simulink model "velocity_pi_pid_control"  (R2025a)
settings: Solver=ode3  StartTime=0.0  StopTime=10  FixedStep=ts  RelTol=1e-3  EnableMultiTasking=on
undefined symbols (not defined in the file): DiscIntNeverNeededParam, ts
libraries: arduinolib x3, simulink x2, arduinosensorlib x1, dspstat3 x1, dspsrcs4 x1
settings Model: SILPILModeSetting=veronly  ExtModeTrigDuration=2  Creator=tsuga  LastModifiedBy=ANUSHKA
settings SolverCC: AutoInsertRateTranBlk=on
settings DataIOCC: SaveOutput=off  SignalLogging=off  DSMLogging=off  SaveTime=off  ReturnWorkspaceOutputs=off
settings OptimizationCC: StrengthReduction=on  PassReuseOutputArgsAs=Individual arguments  ZeroExternalMemoryAtStartup=off  ZeroInternalMemoryAtStartup=off  MaxStackSize=64  OptimizeBlockOrder=speed  OptimizationPriority=Speed  OptimizationCustomize=off  MultiThreadedLoops=on  AutoScheduleForLoops=on  EfficientTunableParamExpr=on
settings DebuggingCC: ParameterTunabilityLossMsg=error  UnconnectedInputMsg=warning  UnconnectedOutputMsg=warning  UnconnectedLineMsg=warning
settings HardwareCC: ProdBitPerInt=16.0  ProdBitPerPointer=16.0  ProdBitPerSizeT=16.0  ProdBitPerPtrDiffT=16.0  ProdLargestAtomicFloat=None  ProdWordSize=8.0  ProdHWDeviceType=Atmel->AVR
settings ModelReferenceCC: EnableRefExpFcnMdlSchedulingChecks=on
settings SFSimCC: MATLABDynamicMemAlloc=off
settings RTWCC: SystemTargetFile=ert.tlc  HardwareBoard=Arduino Uno  TemplateMakefile=ert_default_tmf  Toolchain=Arduino AVR  BuildConfiguration=Faster Runs  GPUComputeCapability=3.5  DLArmComputeVersion=19.05  Description=Embedded Coder
settings CodeAppCC: ForceParamTrailComments=on  IgnoreCustomStorageClasses=off  OperatorAnnotations=on  SimulinkDataObjDesc=on  SFDataObjDesc=on  InsertBlockDesc=on
settings ERTTargetCC: ExtModeTransport=3.0  ExtModeAutomaticAllocSize=off  ExtModeStaticAllocSize=250.0  InlinedParameterPlacement=Hierarchical  DynamicArrayContainerType=coder::array  SupportContinuousTime=on  SupportVariableSizeSignals=on

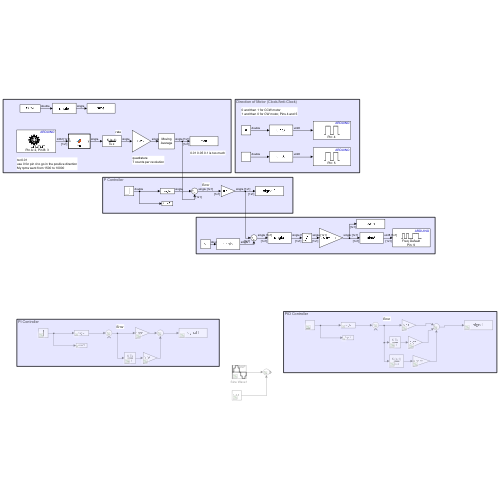
[thumbnail: Simulink's stored preview of the top-level diagram]
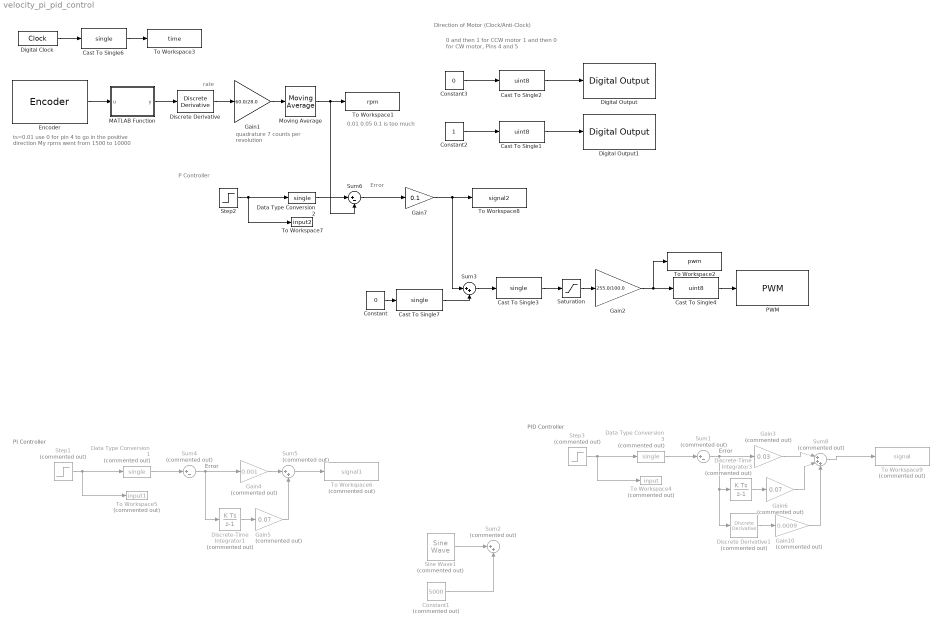
== system velocity_pi_pid_control ==
  note: Direction of Motor (Clock/Anti-Clock)
  note: 0.01 0.05 0.1 is too much
  note: rate
  note: quadrature
      | 7 counts per revolution
  note: ts=0.01
      | use 0 for pin 4 to go in the positive direction
      | My rpms went from 1500 to 10000
  note: 0 and then 1 for CCW motor
      | 1 and then 0 for CW motor, Pins 4 and 5
  note: PI Controller
  note: Error
  note: P Controller
  note: Error
  note: PID Controller
  note: Error
  Cast To Single1 : DataTypeConversion  OutDataTypeStr=uint8  SaturateOnIntegerOverflow=off  RndMeth=Floor
  Cast To Single2 : DataTypeConversion  OutDataTypeStr=uint8  SaturateOnIntegerOverflow=off  RndMeth=Floor
  Cast To Single3 : DataTypeConversion  OutDataTypeStr=single  SaturateOnIntegerOverflow=off  RndMeth=Floor
  Cast To Single4 : DataTypeConversion  OutDataTypeStr=uint8  SaturateOnIntegerOverflow=off  RndMeth=Floor
  Cast To Single6 : DataTypeConversion  OutDataTypeStr=single  SaturateOnIntegerOverflow=off  RndMeth=Floor
  Cast To Single7 : DataTypeConversion  OutDataTypeStr=single  SaturateOnIntegerOverflow=off  RndMeth=Floor
  Constant : Constant  Value=0  SampleTime=ts
  Constant1 : Constant  Commented=on  Value=5000  OutDataTypeStr=double
  Constant2 : Constant  SampleTime=ts
  Constant3 : Constant  Value=0  SampleTime=ts
  Data Type Conversion1 : DataTypeConversion  Commented=on  OutDataTypeStr=single  SaturateOnIntegerOverflow=off  RndMeth=Floor
  Data Type Conversion2 : DataTypeConversion  OutDataTypeStr=single  SaturateOnIntegerOverflow=off  RndMeth=Floor
  Data Type Conversion3 : DataTypeConversion  Commented=on  OutDataTypeStr=single  SaturateOnIntegerOverflow=off  RndMeth=Floor
  Digital Clock : DigitalClock  SampleTime=ts
  Digital Output : arduinolib/Digital Output  pinNumber=4  Direction=output  blockPlatform=arduino
  Digital Output1 : arduinolib/Digital Output  pinNumber=5  Direction=output  blockPlatform=arduino
  Discrete Derivative : simulink/Discrete/Discrete Derivative  gainval=1.0  ICPrevScaledInput=0.0  OutMin=[]  OutMax=[]  OutDataType=fixdt(1, 16)  OutScaling=2^-10  DoSatur=off
  Discrete Derivative1 : simulink/Discrete/Discrete Derivative  Commented=on  gainval=1.0  ICPrevScaledInput=0.0  OutMin=[]  OutMax=[]  OutDataType=fixdt(1, 16)  OutScaling=2^-10  DoSatur=off
  Discrete-Time Integrator1 : DiscreteIntegrator  Commented=on  SampleTime=-1  ICPrevOutput=DiscIntNeverNeededParam  ICPrevScaledInput=DiscIntNeverNeededParam
  Discrete-Time Integrator3 : DiscreteIntegrator  Commented=on  SampleTime=-1  ICPrevOutput=DiscIntNeverNeededParam  ICPrevScaledInput=DiscIntNeverNeededParam
  Encoder : arduinosensorlib/Encoder  InputA=2  InputB=3  Mode=No reset  SampleTime=ts
  Gain1 : Gain  Gain=60.0/28.0
  Gain10 : Gain  Commented=on  Gain=0.0009
  Gain2 : Gain  Gain=255.0/100.0
  Gain3 : Gain  Commented=on  Gain=0.03
  Gain4 : Gain  Commented=on  Gain=0.001
  Gain5 : Gain  Commented=on  Gain=0.07
  Gain6 : Gain  Commented=on  Gain=0.07
  Gain7 : Gain  Gain=0.1
  MATLAB Function : MATLAB Function  TreatAsAtomicUnit=on
  Moving Average : dspstat3/Moving Average  Method=Sliding window  ForgettingFactorPort=off  SpecifyWindowLength=on  WindowLength=8  OverlapLength=7  AllowArbitraryInputLength=off  ForgettingFactor=0.9  SimulateUsing=Code generation
  PWM : arduinolib/PWM  pinNumber=9  frequencyType=Default  desiredFrequency=490.2  achievableFrequency=490.2
  Saturation : Saturate  UpperLimit=100  LowerLimit=0
  Sine Wave1 : dspsrcs4/Sine Wave  Commented=on  Amplitude=3000  Frequency=0.2  Phase=0  SampleMode=Discrete  OutComplex=Real  CompMethod=Trigonometric fcn  TableSize=Speed  SampleTime=ts  SamplesPerFrame=1  ResetState=Restart at time zero  OutputFrames=off  dataType=double  wordLen=16  udDataType=sfix(16)  fracBitsMode=Best precision  numFracBits=15  OutDataTypeStr=double  LastOutDataTypeStr=double
  Step1 : Step  Commented=on  After=5000  SampleTime=0
  Step2 : Step  After=5000  SampleTime=0
  Step3 : Step  Commented=on  After=5000  SampleTime=0
  Sum1 : Sum  Commented=on  Inputs=|+-
  Sum2 : Sum  Commented=on  Inputs=|++
  Sum3 : Sum  Inputs=|++
  Sum4 : Sum  Commented=on  Inputs=|+-
  Sum5 : Sum  Commented=on  Inputs=|++
  Sum6 : Sum  Inputs=|+-
  Sum8 : Sum  Commented=on  Inputs=|+++
  To Workspace1 : ToWorkspace  VariableName=rpm  SampleTime=ts
      settings: Save2DSignal=2-D array (concatenate along first dimension)
  To Workspace2 : ToWorkspace  VariableName=pwm  SampleTime=ts
      settings: Save2DSignal=2-D array (concatenate along first dimension)
  To Workspace3 : ToWorkspace  VariableName=time  SampleTime=ts
      settings: Save2DSignal=2-D array (concatenate along first dimension)
  To Workspace4 : ToWorkspace  Commented=on  VariableName=input  SampleTime=-1
  To Workspace5 : ToWorkspace  Commented=on  VariableName=input1  SampleTime=-1
  To Workspace6 : ToWorkspace  Commented=on  VariableName=signal1  SampleTime=ts
      settings: Save2DSignal=2-D array (concatenate along first dimension)
  To Workspace7 : ToWorkspace  VariableName=input2  SampleTime=-1
  To Workspace8 : ToWorkspace  VariableName=signal2  SampleTime=ts
      settings: Save2DSignal=2-D array (concatenate along first dimension)
  To Workspace9 : ToWorkspace  Commented=on  VariableName=signal  SampleTime=ts
      settings: Save2DSignal=2-D array (concatenate along first dimension)
  wires:
  Cast To Single3/1 -> Saturation/1
  Saturation/1 -> Gain2/1
  Gain2/1 -> Cast To Single4/1, To Workspace2/1
  Cast To Single4/1 -> PWM/1
  Constant2/1 -> Cast To Single1/1
  Cast To Single1/1 -> Digital Output1/1
  Cast To Single2/1 -> Digital Output/1
  Constant3/1 -> Cast To Single2/1
  MATLAB Function/1(y) -> Discrete Derivative/1
  Sum3/1 -> Cast To Single3/1
  Constant/1 -> Cast To Single7/1
  Encoder/1 -> MATLAB Function/1(u)
  Discrete Derivative/1 -> Gain1/1
  Gain1/1 -> Moving Average/1
  Moving Average/1 -> Sum6/2, To Workspace1/1
  Digital Clock/1 -> Cast To Single6/1
  Cast To Single6/1 -> To Workspace3/1
  Cast To Single7/1 -> Sum3/2
  Constant1/1 -> Sum2/2
  Sine Wave1/1 -> Sum2/1
  Discrete-Time Integrator1/1 -> Gain5/1
  Gain5/1 -> Sum5/2
  Data Type Conversion1/1 -> Sum4/1
  Step1/1 -> To Workspace5/1, Data Type Conversion1/1
  Gain4/1 -> Sum5/1
  Sum4/1 -> Discrete-Time Integrator1/1, Gain4/1
  Sum5/1 -> To Workspace6/1
  Data Type Conversion2/1 -> Sum6/1
  Step2/1 -> To Workspace7/1, Data Type Conversion2/1
  Sum6/1 -> Gain7/1
  Gain7/1 -> Sum3/1, To Workspace8/1
  Sum1/1 -> Discrete Derivative1/1, Discrete-Time Integrator3/1, Gain3/1
  Gain3/1 -> Sum8/1
  Sum8/1 -> To Workspace9/1
  Gain6/1 -> Sum8/2
  Discrete-Time Integrator3/1 -> Gain6/1
  Discrete Derivative1/1 -> Gain10/1
  Step3/1 -> To Workspace4/1, Data Type Conversion3/1
  Gain10/1 -> Sum8/3
  Data Type Conversion3/1 -> Sum1/1

== matlab function velocity_pi_pid_control/MATLAB Function ==
  data: u input; y output
function y = fcn(u)
%#codegen

% xx = typecast(u,'single');
% y=xx(1);

y=single(u);  % this method worked
